simulink model "stepc_e"  (R2021b)
settings: Solver=VariableStepAuto  StartTime=0.0  StopTime=10.0  RelTol=1e-3
settings Model: Creator=mustafaenesozdel  LastModifiedBy=emirhankilic
settings DebuggingCC: UnconnectedInputMsg=none  UnconnectedOutputMsg=none  UnconnectedLineMsg=none
settings ModelReferenceCC: EnableRefExpFcnMdlSchedulingChecks=off
settings RTWCC: GPUComputeCapability=5.0  DLArmComputeVersion=20.02.1

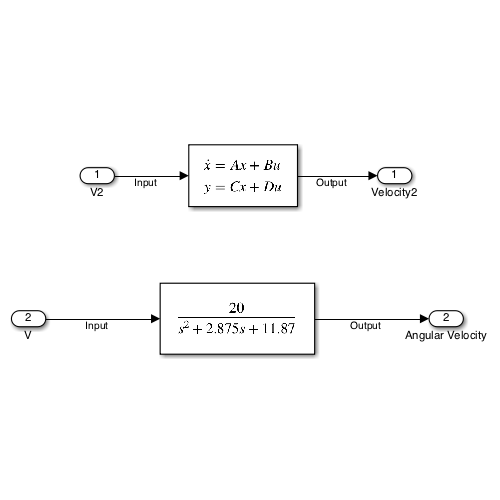
[thumbnail: Simulink's stored preview of the top-level diagram]
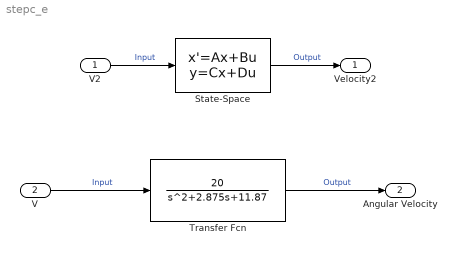
== system stepc_e ==
  V2 : Inport
  V : Inport  Port=2
  State-Space : StateSpace  A=[-1 16; -0.625 -1.875]  B=[0; 1.25]  C=[1 0]  D=0  InitialCondition=0  ContinuousStateAttributes='velocity'
  Transfer Fcn : TransferFcn  Numerator=[20]  Denominator=[1 2.875 11.87]
  Velocity2 : Outport
  Angular Velocity : Outport  Port=2
  wires:
  V2/1 -> State-Space/1  "Input"
  State-Space/1 -> Velocity2/1  "Output"
  Transfer Fcn/1 -> Angular Velocity/1  "Output"
  V/1 -> Transfer Fcn/1  "Input"
